simulink model "sim_tvt_2025_pos_ctrl"  (R2020a)
settings: Solver=ode4  StartTime=0.0  StopTime=30.0  FixedStep=0.01  RelTol=1e-3
values from neighbouring files (symbols this model uses):
  alfa = 0.02    [init_tvt_2025_pos_ctrl.m]
  alfa_theta = 20    [init_tvt_2025_pos_ctrl.m]
  alfa_theta_obs = 100    [init_tvt_2025_pos_ctrl.m]
  c0 = 0.1    [init_tvt_2025_pos_ctrl.m]
  c1_diff_sigma_bar_v = diag([25; 30; 20])    [init_tvt_2025_pos_ctrl.m]
  c1v = diag([5.8; 6.5; 6.5])    [init_tvt_2025_pos_ctrl.m]
  c2_diff_sigma_bar_v = diag([50; 50; 10])    [init_tvt_2025_pos_ctrl.m]
  c2v = diag([5.8; 6.5; 6.5])    [init_tvt_2025_pos_ctrl.m]
  c3_diff_sigma_bar_v = diag([15; 15; 10])    [init_tvt_2025_pos_ctrl.m]
  c3v = diag([4.8; 6.4; 6.0])    [init_tvt_2025_pos_ctrl.m]
  delta_p_i_0 = zeros(3, NF)    [init_tvt_2025_pos_ctrl.m]
  delta_v_i_0 = zeros(3, NF)    [init_tvt_2025_pos_ctrl.m]
  dp_aa_t = 0.2 * ones(3, 5) + ( 1.0 - 0.2 ) * rand(3, 5)    [init_tvt_2025_pos_ctrl.m]
  dp_ff_t = [ 0.4 * ones(1, 5) + ( 1.0 - 0.4 ) * rand(1, 5);                      0.4 * ones(1, 5) + ( 1.0 - 0.4 ) * rand(1, 5);                      0.2 * ones(1, 5) + ( 0.6 - 0.2 ) * rand(1, 5) ]    [init_tvt_2025_pos_ctrl.m]
  dp_phi_t = ( - pi / 2 ) * ones(3, 5) + ( pi / 2 - ( - pi / 2 ) ) * rand(3, 5)    [init_tvt_2025_pos_ctrl.m]
  eps0 = [0.05; 0.01; 0.01]    [init_tvt_2025_pos_ctrl.m]
  eta_ld_hat_init = zeros(3,NF)    [init_tvt_2025_pos_ctrl.m]
  etai_0 = zeros(3,5)    [init_tvt_2025_pos_ctrl.m]
  gamma0 = diag([1, 1, 1])    [init_tvt_2025_pos_ctrl.m]
  k_phi = diag([10, 10, 10])    [init_tvt_2025_pos_ctrl.m]
  k_theta = diag([5, 5, 5])    [init_tvt_2025_pos_ctrl.m]
  kai0 = [15; 10; 10]    [init_tvt_2025_pos_ctrl.m]
  kai_1_t = 0.02    [init_tvt_2025_pos_ctrl.m]
  kai_3_t = 0.1    [init_tvt_2025_pos_ctrl.m]
  ksi_ld_hat_init = zeros(3,NF)    [init_tvt_2025_pos_ctrl.m]
  ksii_0 = zeros(3,5)    [init_tvt_2025_pos_ctrl.m]
  l1v = diag([20; 20; 20])    [init_tvt_2025_pos_ctrl.m]
  l2v = diag([30; 30; 30])    [init_tvt_2025_pos_ctrl.m]
  lam0 = [15; 10; 10]    [init_tvt_2025_pos_ctrl.m]
  lam1 = diag([5,5,5])    [init_tvt_2025_pos_ctrl.m]
  lam2 = diag([5,5,5])    [init_tvt_2025_pos_ctrl.m]
  lam3 = diag([5,5,5])    [init_tvt_2025_pos_ctrl.m]
  lam4 = diag([5,5,5])    [init_tvt_2025_pos_ctrl.m]
  Lamd_diff_sigma_bar_v = 0.5    [init_tvt_2025_pos_ctrl.m]
  mass_i = zeros(1,NF)    [init_tvt_2025_pos_ctrl.m]
  Mii = diag([1;0;0;0;1])    [init_tvt_2025_pos_ctrl.m]
  pos0 = zeros(3, 1)    [init_tvt_2025_pos_ctrl.m]
  pos_bar_init = zeros(3,NF)    [init_tvt_2025_pos_ctrl.m]
  PZ0 = P0(3)    [init_tvt_2025_pos_ctrl.m]
  PZ1 = 10    [init_tvt_2025_pos_ctrl.m]
  Qci_init = repmat([1;0;0;0],1,NF)    [init_tvt_2025_pos_ctrl.m]
  R0 = 4    [init_tvt_2025_pos_ctrl.m]
  R1 = 8    [init_tvt_2025_pos_ctrl.m]
  Rx2 = 10    [init_tvt_2025_pos_ctrl.m]
  Ry2 = 6    [init_tvt_2025_pos_ctrl.m]
  Rz2 = 4    [init_tvt_2025_pos_ctrl.m]
  T0 = 0    [init_tvt_2025_pos_ctrl.m]
  T1 = tseq1    (= 10)    [init_tvt_2025_pos_ctrl.m]
  T12 = tseq1 + tseq12    (= 20)    [init_tvt_2025_pos_ctrl.m]
  T2 = tseq1 + tseq12 + tseq2    (= 30)    [init_tvt_2025_pos_ctrl.m]
  theta0 = ( 2 / 5 ) * pi    (= 1.25663706144)    [init_tvt_2025_pos_ctrl.m]
  vel0 = zeros(3, 1)    [init_tvt_2025_pos_ctrl.m]
  vel_bar_init = zeros(3,NF)    [init_tvt_2025_pos_ctrl.m]
  Wij = [0,0,1,0,0;              0,0,1,1,0;              1,0,0,0,1;              0,1,1,0,0;              0,0,1,0,0]    [init_tvt_2025_pos_ctrl.m]
  X1 = 8    [init_tvt_2025_pos_ctrl.m]
  X2 = 2    [init_tvt_2025_pos_ctrl.m]
  X3 = 3    [init_tvt_2025_pos_ctrl.m]
  Y1 = 10    [init_tvt_2025_pos_ctrl.m]
  Y2 = 2    [init_tvt_2025_pos_ctrl.m]
  Y3 = 4    [init_tvt_2025_pos_ctrl.m]
  Z1 = 4    [init_tvt_2025_pos_ctrl.m]
  Z2 = -6    [init_tvt_2025_pos_ctrl.m]
  Z3 = 2    [init_tvt_2025_pos_ctrl.m]
  zeta_diff_sigma_bar_v = 0.08    [init_tvt_2025_pos_ctrl.m]
undefined symbols (not defined in the file or in its folder): cal_frac_squ, p_alfav1, p_alfav2, p_gamma1_pos, p_gamma1_vel, p_gamma2_pos, p_gamma2_vel, q_alfav1, q_alfav2, q_gamma1_pos, q_gamma1_vel, q_gamma2_pos, q_gamma2_vel
(part 5 of 5)

== matlab function sim_tvt_2025_pos_ctrl/combine lumped follower position observation error ==
  data: theta_ksi_est_err_tilt_1_1 input; theta_ksi_est_err_tilt_1_2 input; theta_ksi_est_err_tilt_1_3 input; theta_ksi_est_err_tilt_1_4 input; theta_ksi_est_err_tilt_1_5 input; theta_ksi_est_err_tilt_1_vec output; theta_ksi_est_err_tilt_2_1 input; theta_ksi_est_err_tilt_2_vec output; theta_ksi_est_err_tilt_2_2 input; theta_ksi_est_err_tilt_2_3 input; theta_ksi_est_err_tilt_2_4 input; theta_ksi_est_err_tilt_2_5 input
function [theta_ksi_est_err_tilt_1_vec, theta_ksi_est_err_tilt_2_vec]  = fcn(theta_ksi_est_err_tilt_1_1, theta_ksi_est_err_tilt_1_2, theta_ksi_est_err_tilt_1_3, theta_ksi_est_err_tilt_1_4, theta_ksi_est_err_tilt_1_5, ...
                                                                                                                                    theta_ksi_est_err_tilt_2_1, theta_ksi_est_err_tilt_2_2, theta_ksi_est_err_tilt_2_3, theta_ksi_est_err_tilt_2_4, theta_ksi_est_err_tilt_2_5)
%%%% 合并领导者位置观测器输出结果
theta_ksi_est_err_tilt_1_vec = [theta_ksi_est_err_tilt_1_1(:), theta_ksi_est_err_tilt_1_2(:), theta_ksi_est_err_tilt_1_3(:), theta_ksi_est_err_tilt_1_4(:), theta_ksi_est_err_tilt_1_5(:)];
theta_ksi_est_err_tilt_2_vec = [theta_ksi_est_err_tilt_2_1(:), theta_ksi_est_err_tilt_2_2(:), theta_ksi_est_err_tilt_2_3(:), theta_ksi_est_err_tilt_2_4(:), theta_ksi_est_err_tilt_2_5(:)];

== matlab function sim_tvt_2025_pos_ctrl/cal rho_err_vec ==
  data: u0 input; rho_err_vec output; rho_hat_vec input
function rho_err_vec  = fcn(u0, rho_hat_vec)
%%%% 计算分布式观测误差
rho_err_vec = zeros(3,5);
for iiuav = 1:5
    rho_err_vec(:,iiuav) = u0(:) - rho_hat_vec(:,iiuav);
end

== matlab function sim_tvt_2025_pos_ctrl/combine lumped follower velocity observation error ==
  data: theta_eta_est_err_tilt_1_1 input; theta_eta_est_err_tilt_1_2 input; theta_eta_est_err_tilt_1_3 input; theta_eta_est_err_tilt_1_4 input; theta_eta_est_err_tilt_1_5 input; theta_eta_est_err_tilt_1_vec output; theta_eta_est_err_tilt_2_1 input; theta_eta_est_err_tilt_2_vec output; theta_eta_est_err_tilt_2_2 input; theta_eta_est_err_tilt_2_3 input; theta_eta_est_err_tilt_2_4 input; theta_eta_est_err_tilt_2_5 input
function [theta_eta_est_err_tilt_1_vec, theta_eta_est_err_tilt_2_vec]  = fcn(theta_eta_est_err_tilt_1_1, theta_eta_est_err_tilt_1_2, theta_eta_est_err_tilt_1_3, theta_eta_est_err_tilt_1_4, theta_eta_est_err_tilt_1_5, ...
                                                                                                                                    theta_eta_est_err_tilt_2_1, theta_eta_est_err_tilt_2_2, theta_eta_est_err_tilt_2_3, theta_eta_est_err_tilt_2_4, theta_eta_est_err_tilt_2_5)
%%%% 合并领导者位置观测器输出结果
theta_eta_est_err_tilt_1_vec = [theta_eta_est_err_tilt_1_1(:), theta_eta_est_err_tilt_1_2(:), theta_eta_est_err_tilt_1_3(:), theta_eta_est_err_tilt_1_4(:), theta_eta_est_err_tilt_1_5(:)];
theta_eta_est_err_tilt_2_vec = [theta_eta_est_err_tilt_2_1(:), theta_eta_est_err_tilt_2_2(:), theta_eta_est_err_tilt_2_3(:), theta_eta_est_err_tilt_2_4(:), theta_eta_est_err_tilt_2_5(:)];

== matlab function sim_tvt_2025_pos_ctrl/fixed-time distributed follower desire position observer agent 1 ==
  data: l1p input; d_ksi_d_est_1 output; l2p input; eta_d_est_vec input; theta_ksi_est_err_tilt_1_vec input; theta_ksi_est_err_tilt_2_vec input
function d_ksi_d_est_1 = fcn(l1p, l2p, eta_d_est_vec, theta_ksi_est_err_tilt_1_vec, theta_ksi_est_err_tilt_2_vec)
%%%% 固定时间跟随者期望位置分布式观测器
iiuav = 1;
d_ksi_d_est_1 = eta_d_est_vec(:,iiuav) - l1p * theta_ksi_est_err_tilt_1_vec(:,iiuav) - l2p * theta_ksi_est_err_tilt_2_vec(:,iiuav);

== matlab function sim_tvt_2025_pos_ctrl/fixed-time distributed follower desire position observer agent 2 ==
  data: l1p input; d_ksi_d_est_2 output; l2p input; eta_d_est_vec input; theta_ksi_est_err_tilt_1_vec input; theta_ksi_est_err_tilt_2_vec input
function d_ksi_d_est_2 = fcn(l1p, l2p, eta_d_est_vec, theta_ksi_est_err_tilt_1_vec, theta_ksi_est_err_tilt_2_vec)
%%%% 固定时间跟随者期望位置分布式观测器
iiuav = 2;
d_ksi_d_est_2 = eta_d_est_vec(:,iiuav) - l1p * theta_ksi_est_err_tilt_1_vec(:,iiuav) - l2p * theta_ksi_est_err_tilt_2_vec(:,iiuav);

== matlab function sim_tvt_2025_pos_ctrl/fixed-time distributed follower desire position observer agent 3 ==
  data: l1p input; d_ksi_d_est_3 output; l2p input; eta_d_est_vec input; theta_ksi_est_err_tilt_1_vec input; theta_ksi_est_err_tilt_2_vec input
function d_ksi_d_est_3 = fcn(l1p, l2p, eta_d_est_vec, theta_ksi_est_err_tilt_1_vec, theta_ksi_est_err_tilt_2_vec)
%%%% 固定时间跟随者期望位置分布式观测器
iiuav = 3;
d_ksi_d_est_3 = eta_d_est_vec(:,iiuav) - l1p * theta_ksi_est_err_tilt_1_vec(:,iiuav) - l2p * theta_ksi_est_err_tilt_2_vec(:,iiuav);

== matlab function sim_tvt_2025_pos_ctrl/fixed-time distributed follower desire position observer agent 4 ==
  data: l1p input; d_ksi_d_est_4 output; l2p input; eta_d_est_vec input; theta_ksi_est_err_tilt_1_vec input; theta_ksi_est_err_tilt_2_vec input
function d_ksi_d_est_4 = fcn(l1p, l2p, eta_d_est_vec, theta_ksi_est_err_tilt_1_vec, theta_ksi_est_err_tilt_2_vec)
%%%% 固定时间跟随者期望位置分布式观测器
iiuav = 4;
d_ksi_d_est_4 = eta_d_est_vec(:,iiuav) - l1p * theta_ksi_est_err_tilt_1_vec(:,iiuav) - l2p * theta_ksi_est_err_tilt_2_vec(:,iiuav);

== matlab function sim_tvt_2025_pos_ctrl/fixed-time distributed follower desire position observer agent 5 ==
  data: l1p input; d_ksi_d_est_5 output; l2p input; eta_d_est_vec input; theta_ksi_est_err_tilt_1_vec input; theta_ksi_est_err_tilt_2_vec input
function d_ksi_d_est_5 = fcn(l1p, l2p, eta_d_est_vec, theta_ksi_est_err_tilt_1_vec, theta_ksi_est_err_tilt_2_vec)
%%%% 固定时间跟随者期望位置分布式观测器
iiuav = 5;
d_ksi_d_est_5 = eta_d_est_vec(:,iiuav) - l1p * theta_ksi_est_err_tilt_1_vec(:,iiuav) - l2p * theta_ksi_est_err_tilt_2_vec(:,iiuav);

== matlab function sim_tvt_2025_pos_ctrl/fixed-time distributed follower desire velocity observer agent 1 ==
  data: l1v input; d_eta_d_est_1 output; l2v input; theta_eta_est_err_tilt_1_vec input; theta_eta_est_err_tilt_2_vec input
function d_eta_d_est_1 = fcn(l1v, l2v, theta_eta_est_err_tilt_1_vec, theta_eta_est_err_tilt_2_vec)
%%%% 固定时间跟随者期望速度分布式观测器
iiuav = 1;
d_eta_d_est_1 = -l1v * theta_eta_est_err_tilt_1_vec(:,iiuav) - l2v * theta_eta_est_err_tilt_2_vec(:,iiuav);

== matlab function sim_tvt_2025_pos_ctrl/cal abs 41 ==
  data: x input; y output
function y = fcn(x)
y = abs(x(:));

== matlab function sim_tvt_2025_pos_ctrl/fixed-time distributed follower desire velocity observer agent 2 ==
  data: l1v input; d_eta_d_est_2 output; l2v input; theta_eta_est_err_tilt_1_vec input; theta_eta_est_err_tilt_2_vec input
function d_eta_d_est_2 = fcn(l1v, l2v, theta_eta_est_err_tilt_1_vec, theta_eta_est_err_tilt_2_vec)
%%%% 固定时间跟随者期望速度分布式观测器
iiuav = 2;
d_eta_d_est_2 = -l1v * theta_eta_est_err_tilt_1_vec(:,iiuav) - l2v * theta_eta_est_err_tilt_2_vec(:,iiuav);

== matlab function sim_tvt_2025_pos_ctrl/fixed-time distributed follower desire velocity observer agent 3 ==
  data: l1v input; d_eta_d_est_3 output; l2v input; theta_eta_est_err_tilt_1_vec input; theta_eta_est_err_tilt_2_vec input
function d_eta_d_est_3 = fcn(l1v, l2v, theta_eta_est_err_tilt_1_vec, theta_eta_est_err_tilt_2_vec)
%%%% 固定时间跟随者期望速度分布式观测器
iiuav = 3;
d_eta_d_est_3 = -l1v * theta_eta_est_err_tilt_1_vec(:,iiuav) - l2v * theta_eta_est_err_tilt_2_vec(:,iiuav);

== matlab function sim_tvt_2025_pos_ctrl/fixed-time distributed follower desire velocity observer agent 4 ==
  data: l1v input; d_eta_d_est_4 output; l2v input; theta_eta_est_err_tilt_1_vec input; theta_eta_est_err_tilt_2_vec input
function d_eta_d_est_4 = fcn(l1v, l2v, theta_eta_est_err_tilt_1_vec, theta_eta_est_err_tilt_2_vec)
%%%% 固定时间跟随者期望速度分布式观测器
iiuav = 4;
d_eta_d_est_4 = -l1v * theta_eta_est_err_tilt_1_vec(:,iiuav) - l2v * theta_eta_est_err_tilt_2_vec(:,iiuav);

== matlab function sim_tvt_2025_pos_ctrl/fixed-time distributed follower desire velocity observer agent 5 ==
  data: l1v input; d_eta_d_est_5 output; l2v input; theta_eta_est_err_tilt_1_vec input; theta_eta_est_err_tilt_2_vec input
function d_eta_d_est_5 = fcn(l1v, l2v, theta_eta_est_err_tilt_1_vec, theta_eta_est_err_tilt_2_vec)
%%%% 固定时间跟随者期望速度分布式观测器
iiuav = 5;
d_eta_d_est_5 = -l1v * theta_eta_est_err_tilt_1_vec(:,iiuav) - l2v * theta_eta_est_err_tilt_2_vec(:,iiuav);

== matlab function sim_tvt_2025_pos_ctrl/trans to column41 ==
  data: x input; y output
function y = fcn(x)
y = x(:);

== matlab function sim_tvt_2025_pos_ctrl/trans to column42 ==
  data: x input; y output
function y = fcn(x)
y = x(:);

== matlab function sim_tvt_2025_pos_ctrl/trans to column43 ==
  data: x input; y output
function y = fcn(x)
y = x(:);

== matlab function sim_tvt_2025_pos_ctrl/trans to column44 ==
  data: x input; y output
function y = fcn(x)
y = x(:);

== matlab function sim_tvt_2025_pos_ctrl/cal abs 42 ==
  data: x input; y output
function y = fcn(x)
y = abs(x(:));

== matlab function sim_tvt_2025_pos_ctrl/trans to column45 ==
  data: x input; y output
function y = fcn(x)
y = x(:);

== matlab function sim_tvt_2025_pos_ctrl/trans to column46 ==
  data: x input; y output
function y = fcn(x)
y = x(:);

== matlab function sim_tvt_2025_pos_ctrl/trans to column47 ==
  data: x input; y output
function y = fcn(x)
y = x(:);

== matlab function sim_tvt_2025_pos_ctrl/trans to column48 ==
  data: x input; y output
function y = fcn(x)
y = x(:);

== matlab function sim_tvt_2025_pos_ctrl/trans to column49 ==
  data: x input; y output
function y = fcn(x)
y = x(:);

== matlab function sim_tvt_2025_pos_ctrl/trans to column50 ==
  data: x input; y output
function y = fcn(x)
y = x(:);

== matlab function sim_tvt_2025_pos_ctrl/trans to column51 ==
  data: x input; y output
function y = fcn(x)
y = x(:);

== matlab function sim_tvt_2025_pos_ctrl/trans to column52 ==
  data: x input; y output
function y = fcn(x)
y = x(:);

== matlab function sim_tvt_2025_pos_ctrl/trans to column53 ==
  data: x input; y output
function y = fcn(x)
y = x(:);

== matlab function sim_tvt_2025_pos_ctrl/trans to column54 ==
  data: x input; y output
function y = fcn(x)
y = x(:);

== matlab function sim_tvt_2025_pos_ctrl/cal abs 43 ==
  data: x input; y output
function y = fcn(x)
y = abs(x(:));

== matlab function sim_tvt_2025_pos_ctrl/trans to column55 ==
  data: x input; y output
function y = fcn(x)
y = x(:);

== matlab function sim_tvt_2025_pos_ctrl/trans to column56 ==
  data: x input; y output
function y = fcn(x)
y = x(:);

== matlab function sim_tvt_2025_pos_ctrl/trans to column57 ==
  data: x input; y output
function y = fcn(x)
y = x(:);

== matlab function sim_tvt_2025_pos_ctrl/trans to column58 ==
  data: x input; y output
function y = fcn(x)
y = x(:);

== matlab function sim_tvt_2025_pos_ctrl/trans to column59 ==
  data: x input; y output
function y = fcn(x)
y = x(:);

== matlab function sim_tvt_2025_pos_ctrl/trans to column60 ==
  data: x input; y output
function y = fcn(x)
y = x(:);

== matlab function sim_tvt_2025_pos_ctrl/cal abs 44 ==
  data: x input; y output
function y = fcn(x)
y = abs(x(:));

== matlab function sim_tvt_2025_pos_ctrl/cal abs 45 ==
  data: x input; y output
function y = fcn(x)
y = abs(x(:));

== matlab function sim_tvt_2025_pos_ctrl/cal ui agent 2 ==
  data: k_phi input; rho_hat_vec input; phi_vec input; d_phi_vec input; ui_2 output; dp_hat_vec input
function ui_2 = fcn(k_phi, rho_hat_vec, phi_vec, d_phi_vec, dp_hat_vec)
%%%% 计算控制输入ui
iiuav = 2;
g0 = 9.80663;
e3 = [0;0;1];
ui_2 = g0 * e3 + rho_hat_vec(:,iiuav) - dp_hat_vec(:,iiuav) ...
            - k_phi * ( tanh( phi_vec(:,iiuav) ) + tanh( d_phi_vec(:,iiuav) ) );

== matlab function sim_tvt_2025_pos_ctrl/cal ui agent 3 ==
  data: k_phi input; rho_hat_vec input; phi_vec input; d_phi_vec input; ui_3 output; dp_hat_vec input
function ui_3 = fcn(k_phi, rho_hat_vec, phi_vec, d_phi_vec, dp_hat_vec)
%%%% 计算控制输入ui
iiuav = 3;
g0 = 9.80663;
e3 = [0;0;1];
ui_3 = g0 * e3 + rho_hat_vec(:,iiuav) - dp_hat_vec(:,iiuav) ...
            - k_phi * ( tanh( phi_vec(:,iiuav) ) + tanh( d_phi_vec(:,iiuav) ) );

== matlab function sim_tvt_2025_pos_ctrl/cal ui agent 4 ==
  data: k_phi input; rho_hat_vec input; phi_vec input; d_phi_vec input; ui_4 output; dp_hat_vec input
function ui_4 = fcn(k_phi, rho_hat_vec, phi_vec, d_phi_vec, dp_hat_vec)
%%%% 计算控制输入ui
iiuav = 4;
g0 = 9.80663;
e3 = [0;0;1];
ui_4 = g0 * e3 + rho_hat_vec(:,iiuav) - dp_hat_vec(:,iiuav) ...
            - k_phi * ( tanh( phi_vec(:,iiuav) ) + tanh( d_phi_vec(:,iiuav) ) );

== matlab function sim_tvt_2025_pos_ctrl/cal ui agent 5 ==
  data: k_phi input; rho_hat_vec input; phi_vec input; d_phi_vec input; ui_5 output; dp_hat_vec input
function ui_5 = fcn(k_phi, rho_hat_vec, phi_vec, d_phi_vec, dp_hat_vec)
%%%% 计算控制输入ui
iiuav = 5;
g0 = 9.80663;
e3 = [0;0;1];
ui_5 = g0 * e3 + rho_hat_vec(:,iiuav) - dp_hat_vec(:,iiuav) ...
            - k_phi * ( tanh( phi_vec(:,iiuav) ) + tanh( d_phi_vec(:,iiuav) ) );

== matlab function sim_tvt_2025_pos_ctrl/cal abs 46 ==
  data: x input; y output
function y = fcn(x)
y = abs(x(:));

== matlab function sim_tvt_2025_pos_ctrl/combine formation control input ==
  data: eta_i_vec output; ksi_i_vec output; eta_1 input; eta_2 input; eta_3 input; eta_4 input; eta_5 input; ksi_1 input; ksi_2 input; ksi_3 input; ksi_4 input; ksi_5 input
function [eta_i_vec, ksi_i_vec] = fcn(eta_1, eta_2, eta_3, eta_4, eta_5, ...
                                                                ksi_1, ksi_2, ksi_3, ksi_4, ksi_5)
%%%% 合并领导者编队跟踪误差结果
eta_i_vec = [eta_1(:), eta_2(:), eta_3(:), eta_4(:), eta_5(:)];
ksi_i_vec = [ksi_1(:), ksi_2(:), ksi_3(:), ksi_4(:), ksi_5(:)];

== matlab function sim_tvt_2025_pos_ctrl/cal abs 47 ==
  data: x input; y output
function y = fcn(x)
y = abs(x(:));

== matlab function sim_tvt_2025_pos_ctrl/cal abs 48 ==
  data: x input; y output
function y = fcn(x)
y = abs(x(:));

== matlab function sim_tvt_2025_pos_ctrl/cal abs 49 ==
  data: x input; y output
function y = fcn(x)
y = abs(x(:));

== matlab function sim_tvt_2025_pos_ctrl/cal abs 50 ==
  data: x input; y output
function y = fcn(x)
y = abs(x(:));

== matlab function sim_tvt_2025_pos_ctrl/uav translational dynamics agent 1 ==
  data: dvi output; Ri input; ui input; dpi_vec input
function dvi = fcn(Ri, ui, dpi_vec)
%%%% 根据有限时间控制输入计算无人机平移动力学微分方程
iiuav = 1;
g0 = 9.80663;
e3 = [0;0;1];
dvi = -g0 * e3 + norm(ui(:,iiuav),2) * Ri(:,:,iiuav) * e3 + dpi_vec(:,iiuav);

== matlab function sim_tvt_2025_pos_ctrl/uav translational dynamics agent 2 ==
  data: dvi output; Ri input; ui input; dpi_vec input
function dvi = fcn(Ri, ui, dpi_vec)
%%%% 根据有限时间控制输入计算无人机平移动力学微分方程
iiuav = 2;
g0 = 9.80663;
e3 = [0;0;1];
dvi = -g0 * e3 + norm(ui(:,iiuav),2) * Ri(:,:,iiuav) * e3 + dpi_vec(:,iiuav);

== matlab function sim_tvt_2025_pos_ctrl/uav translational dynamics agent 3 ==
  data: dvi output; Ri input; ui input; dpi_vec input
function dvi = fcn(Ri, ui, dpi_vec)
%%%% 根据有限时间控制输入计算无人机平移动力学微分方程
iiuav = 3;
g0 = 9.80663;
e3 = [0;0;1];
dvi = -g0 * e3 + norm(ui(:,iiuav),2) * Ri(:,:,iiuav) * e3 + dpi_vec(:,iiuav);

== matlab function sim_tvt_2025_pos_ctrl/uav translational dynamics agent 4 ==
  data: dvi output; Ri input; ui input; dpi_vec input
function dvi = fcn(Ri, ui, dpi_vec)
%%%% 根据有限时间控制输入计算无人机平移动力学微分方程
iiuav = 4;
g0 = 9.80663;
e3 = [0;0;1];
dvi = -g0 * e3 + norm(ui(:,iiuav),2) * Ri(:,:,iiuav) * e3 + dpi_vec(:,iiuav);

== matlab function sim_tvt_2025_pos_ctrl/uav translational dynamics agent 5 ==
  data: dvi output; Ri input; ui input; dpi_vec input
function dvi = fcn(Ri, ui, dpi_vec)
%%%% 根据有限时间控制输入计算无人机平移动力学微分方程
iiuav = 5;
g0 = 9.80663;
e3 = [0;0;1];
dvi = -g0 * e3 + norm(ui(:,iiuav),2) * Ri(:,:,iiuav) * e3 + dpi_vec(:,iiuav);

== matlab function sim_tvt_2025_pos_ctrl/cal Ri ==
  data: Ri output; Rei input; Rci input
function Ri = fcn(Rei, Rci)
%%%% 使用罗德里格公式由四元数Qci求解Rci
Ri = zeros(3,3,5);
for iiuav = 1:5
    Ri(:,:,iiuav) = Rci(:,:,iiuav) * Rei(:,:,iiuav);
end

end

== matlab function sim_tvt_2025_pos_ctrl/follower tracking error agent 1 ==
  data: ksi_track_err_1 output; delta_ksi_vec input; delta_eta_vec input; ksi_i_vec input; eta_i_vec input; ksi0 input; eta_track_err_1 output; eta0 input
function [ksi_track_err_1, eta_track_err_1]  = fcn(delta_ksi_vec, delta_eta_vec, ksi_i_vec, eta_i_vec, ksi0, eta0)
%%%% 计算跟随者节点1号位置/速度跟踪误差
eta_track_err_1 = eta_i_vec(:,1) - delta_eta_vec(:,1) - eta0;
ksi_track_err_1 = ksi_i_vec(:,1) - delta_ksi_vec(:,1) - ksi0;

== matlab function sim_tvt_2025_pos_ctrl/follower tracking error agent 2 ==
  data: ksi_track_err_2 output; delta_ksi_vec input; delta_eta_vec input; ksi_i_vec input; eta_i_vec input; ksi0 input; eta_track_err_2 output; eta0 input
function [ksi_track_err_2, eta_track_err_2]  = fcn(delta_ksi_vec, delta_eta_vec, ksi_i_vec, eta_i_vec, ksi0, eta0)
%%%% 计算跟随者节点2号位置/速度跟踪误差
eta_track_err_2 = eta_i_vec(:,2) - delta_eta_vec(:,2) - eta0;
ksi_track_err_2 = ksi_i_vec(:,2) - delta_ksi_vec(:,2) - ksi0;

== matlab function sim_tvt_2025_pos_ctrl/follower tracking error agent 3 ==
  data: ksi_track_err_3 output; delta_ksi_vec input; delta_eta_vec input; ksi_i_vec input; eta_i_vec input; ksi0 input; eta_track_err_3 output; eta0 input
function [ksi_track_err_3, eta_track_err_3]  = fcn(delta_ksi_vec, delta_eta_vec, ksi_i_vec, eta_i_vec, ksi0, eta0)
%%%% 计算跟随者节点3号位置/速度跟踪误差
eta_track_err_3 = eta_i_vec(:,3) - delta_eta_vec(:,3) - eta0;
ksi_track_err_3 = ksi_i_vec(:,3) - delta_ksi_vec(:,3) - ksi0;

== matlab function sim_tvt_2025_pos_ctrl/follower tracking error agent 4 ==
  data: ksi_track_err_4 output; delta_ksi_vec input; delta_eta_vec input; ksi_i_vec input; eta_i_vec input; ksi0 input; eta_track_err_4 output; eta0 input
function [ksi_track_err_4, eta_track_err_4]  = fcn(delta_ksi_vec, delta_eta_vec, ksi_i_vec, eta_i_vec, ksi0, eta0)
%%%% 计算跟随者节点4号位置/速度跟踪误差
eta_track_err_4 = eta_i_vec(:,4) - delta_eta_vec(:,4) - eta0;
ksi_track_err_4 = ksi_i_vec(:,4) - delta_ksi_vec(:,4) - ksi0;

== matlab function sim_tvt_2025_pos_ctrl/follower tracking error agent 5 ==
  data: ksi_track_err_5 output; delta_ksi_vec input; delta_eta_vec input; ksi_i_vec input; eta_i_vec input; ksi0 input; eta_track_err_5 output; eta0 input
function [ksi_track_err_5, eta_track_err_5]  = fcn(delta_ksi_vec, delta_eta_vec, ksi_i_vec, eta_i_vec, ksi0, eta0)
%%%% 计算跟随者节点5号位置/速度跟踪误差
eta_track_err_5 = eta_i_vec(:,5) - delta_eta_vec(:,5) - eta0;
ksi_track_err_5 = ksi_i_vec(:,5) - delta_ksi_vec(:,5) - ksi0;

== matlab function sim_tvt_2025_pos_ctrl/combine follower eta ksi ==
  data: ksi_track_err_vec output; ksi_track_err_1 input; ksi_track_err_2 input; ksi_track_err_3 input; ksi_track_err_4 input; ksi_track_err_5 input; eta_track_err_vec output; eta_track_err_1 input; eta_track_err_2 input; eta_track_err_3 input; eta_track_err_4 input; eta_track_err_5 input
function [ksi_track_err_vec, eta_track_err_vec]  = fcn(ksi_track_err_1, ksi_track_err_2, ksi_track_err_3, ksi_track_err_4, ksi_track_err_5, ...
                                                                                    eta_track_err_1, eta_track_err_2, eta_track_err_3, eta_track_err_4, eta_track_err_5)
%%%% 合并所有跟随者的速度/位置向量
ksi_track_err_vec = [ksi_track_err_1(:), ksi_track_err_2(:), ksi_track_err_3(:), ksi_track_err_4(:), ksi_track_err_5(:)];
eta_track_err_vec = [eta_track_err_1(:), eta_track_err_2(:), eta_track_err_3(:), eta_track_err_4(:), eta_track_err_5(:)];

== matlab function sim_tvt_2025_pos_ctrl/depart Rc5 ==
  data: y output; x input
function y = fcn(x)
y = x(:,:,5);

end

== matlab function sim_tvt_2025_pos_ctrl/depart Rc1 ==
  data: y output; x input
function y = fcn(x)
y = x(:,:,1);

end

== matlab function sim_tvt_2025_pos_ctrl/depart Rc2 ==
  data: y output; x input
function y = fcn(x)
y = x(:,:,2);

end

== matlab function sim_tvt_2025_pos_ctrl/depart Rc3 ==
  data: y output; x input
function y = fcn(x)
y = x(:,:,3);

end

== matlab function sim_tvt_2025_pos_ctrl/depart Rc4 ==
  data: y output; x input
function y = fcn(x)
y = x(:,:,4);

end

== matlab function sim_tvt_2025_pos_ctrl/combine rho_hat ==
  data: rho_hat_1 input; rho_hat_vec output; rho_hat_2 input; rho_hat_3 input; rho_hat_4 input; rho_hat_5 input
function rho_hat_vec  = fcn(rho_hat_1, rho_hat_2, rho_hat_3, rho_hat_4, rho_hat_5)
%%%% 合并领导者加速度分布式观测器
rho_hat_vec = zeros(3,5);
rho_hat_vec(:,1) = rho_hat_1(:);
rho_hat_vec(:,2) = rho_hat_2(:);
rho_hat_vec(:,3) = rho_hat_3(:);
rho_hat_vec(:,4) = rho_hat_4(:);
rho_hat_vec(:,5) = rho_hat_5(:);

== matlab function sim_tvt_2025_pos_ctrl/rho_hat agent 1 ==
  data: lam0 input; rho_hat_1 output; sigmai_vec input
function rho_hat_1 = fcn(lam0, sigmai_vec)
%%%% 领导者加速度分布式观测器
iiuav = 1;
rho_hat_1 = lam0(:) .* tanh( sigmai_vec(:,iiuav) );

== matlab function sim_tvt_2025_pos_ctrl/rho_hat agent 2 ==
  data: lam0 input; rho_hat_2 output; sigmai_vec input
function rho_hat_2 = fcn(lam0, sigmai_vec)
%%%% 领导者加速度分布式观测器
iiuav = 2;
rho_hat_2 = lam0(:) .* tanh( sigmai_vec(:,iiuav) );

== matlab function sim_tvt_2025_pos_ctrl/rho_hat agent 3 ==
  data: lam0 input; rho_hat_3 output; sigmai_vec input
function rho_hat_3 = fcn(lam0, sigmai_vec)
%%%% 领导者加速度分布式观测器
iiuav = 3;
rho_hat_3 = lam0(:) .* tanh( sigmai_vec(:,iiuav) );

== matlab function sim_tvt_2025_pos_ctrl/rho_hat agent 4 ==
  data: lam0 input; rho_hat_4 output; sigmai_vec input
function rho_hat_4 = fcn(lam0, sigmai_vec)
%%%% 领导者加速度分布式观测器
iiuav = 4;
rho_hat_4 = lam0(:) .* tanh( sigmai_vec(:,iiuav) );

== matlab function sim_tvt_2025_pos_ctrl/rho_hat agent 5 ==
  data: lam0 input; rho_hat_5 output; sigmai_vec input
function rho_hat_5 = fcn(lam0, sigmai_vec)
%%%% 领导者加速度分布式观测器
iiuav = 5;
rho_hat_5 = lam0(:) .* tanh( sigmai_vec(:,iiuav) );

== matlab function sim_tvt_2025_pos_ctrl/cal abs 51 ==
  data: x input; y output
function y = fcn(x)
y = abs(x(:));

== matlab function sim_tvt_2025_pos_ctrl/cal abs 52 ==
  data: x input; y output
function y = fcn(x)
y = abs(x(:));

== matlab function sim_tvt_2025_pos_ctrl/cal abs 53 ==
  data: x input; y output
function y = fcn(x)
y = abs(x(:));

== matlab function sim_tvt_2025_pos_ctrl/cal abs 54 ==
  data: x input; y output
function y = fcn(x)
y = abs(x(:));

== matlab function sim_tvt_2025_pos_ctrl/cal abs 55 ==
  data: x input; y output
function y = fcn(x)
y = abs(x(:));

== matlab function sim_tvt_2025_pos_ctrl/cal leader velocity estimate error ==
  data: eta_ld_hat_vec input; eta_ld_est_err output; eta0 input
function eta_ld_est_err  = fcn(eta_ld_hat_vec, eta0)
%%%% 计算领导者速度分布式观测误差
eta_ld_est_err = zeros(3,5);
for iiuav = 1:5
    eta_ld_est_err(:,iiuav) = eta_ld_hat_vec(:,iiuav) - eta0(:);
end

== matlab function sim_tvt_2025_pos_ctrl/cal leader position estimate error ==
  data: ksi_ld_hat_vec input; ksi_ld_est_err output; ksi0 input
function ksi_ld_est_err  = fcn(ksi_ld_hat_vec, ksi0)
%%%% 计算领导者位置分布式观测误差
ksi_ld_est_err = zeros(3,5);
for iiuav = 1:5
    ksi_ld_est_err(:,iiuav) = ksi_ld_hat_vec(:,iiuav) - ksi0(:);
end

== matlab function sim_tvt_2025_pos_ctrl/generate translational disturbance agent 1 ==
  data: dp_aa_t input; dp_ff_t input; dp_phi_t input; dp_1 output; t input
function dp_1 = fcn(dp_aa_t, dp_ff_t, dp_phi_t, t)
%%%% 平移动力学方程中的扰动项设置
epsil_t = zeros(3, 1);

for kk = 1:5
    epsil_t = epsil_t + dp_aa_t(:, kk) .* sin( 2 * pi * dp_ff_t(:, kk) * t + dp_phi_t(:, kk) );
end

dp_1 = [ epsil_t(1) + 1.6 * sin( 0.4 * t ) + 2.0 * cos( 0.5 * t ) + 1.4 * sin( 0.7 * t ) ...
                + 4 * exp( -0.1 * t ) * sin( 0.8 * t ) + 3 / ( 1 + exp( -0.2 * ( t - 15 ) ) ); ...
                epsil_t(2) + 1.2 * sin( 0.2 * t ) + 3 * cos( 0.4 * t ) + 0.8 * sin( 0.6 * t ) ...
                + 2 * exp( -0.15 * t ) * cos( 1.2 * t ) + 3 / ( 1 + exp( -0.3 * ( t - 25 ) ) ); ...
                epsil_t(3) + 1.8 * sin( 0.2 * t ) + 1.6 * sin( 0.3 * t ) + 1.6 * cos( 0.4 * t ) ...
                + 4 * exp( -0.05 * t ) * sin( 0.5 * t + pi / 4 ) + 3 / ( 1 + exp( -0.5 * ( t - 20 ) ) ) ];

== matlab function sim_tvt_2025_pos_ctrl/cal err_pos_i agent 1 ==
  data: delta_ksi_vec input; ksi_i_vec input; ksi_ld_hat_vec input; err_pos_1 output
function err_pos_1 = fcn(delta_ksi_vec, ksi_i_vec, ksi_ld_hat_vec)
%%%% 计算基于分布式观测值的位置跟踪误差
iiuav = 1;
err_pos_1 = ksi_i_vec(:,iiuav) - ksi_ld_hat_vec(:,iiuav) - delta_ksi_vec(:,iiuav);

== matlab function sim_tvt_2025_pos_ctrl/cal err_pos_i agent 2 ==
  data: delta_ksi_vec input; ksi_i_vec input; ksi_ld_hat_vec input; err_pos_2 output
function err_pos_2 = fcn(delta_ksi_vec, ksi_i_vec, ksi_ld_hat_vec)
%%%% 计算基于分布式观测值的位置跟踪误差
iiuav = 2;
err_pos_2 = ksi_i_vec(:,iiuav) - ksi_ld_hat_vec(:,iiuav) - delta_ksi_vec(:,iiuav);

== matlab function sim_tvt_2025_pos_ctrl/cal err_pos_i agent 3 ==
  data: delta_ksi_vec input; ksi_i_vec input; ksi_ld_hat_vec input; err_pos_3 output
function err_pos_3 = fcn(delta_ksi_vec, ksi_i_vec, ksi_ld_hat_vec)
%%%% 计算基于分布式观测值的位置跟踪误差
iiuav = 3;
err_pos_3 = ksi_i_vec(:,iiuav) - ksi_ld_hat_vec(:,iiuav) - delta_ksi_vec(:,iiuav);

== matlab function sim_tvt_2025_pos_ctrl/cal err_pos_i agent 4 ==
  data: delta_ksi_vec input; ksi_i_vec input; ksi_ld_hat_vec input; err_pos_4 output
function err_pos_4 = fcn(delta_ksi_vec, ksi_i_vec, ksi_ld_hat_vec)
%%%% 计算基于分布式观测值的位置跟踪误差
iiuav = 4;
err_pos_4 = ksi_i_vec(:,iiuav) - ksi_ld_hat_vec(:,iiuav) - delta_ksi_vec(:,iiuav);

== matlab function sim_tvt_2025_pos_ctrl/cal err_pos_i agent 5 ==
  data: delta_ksi_vec input; ksi_i_vec input; ksi_ld_hat_vec input; err_pos_5 output
function err_pos_5 = fcn(delta_ksi_vec, ksi_i_vec, ksi_ld_hat_vec)
%%%% 计算基于分布式观测值的位置跟踪误差
iiuav = 5;
err_pos_5 = ksi_i_vec(:,iiuav) - ksi_ld_hat_vec(:,iiuav) - delta_ksi_vec(:,iiuav);

== matlab function sim_tvt_2025_pos_ctrl/combine err_pos_i ==
  data: err_pos_1 input; err_pos_vec output; err_pos_2 input; err_pos_3 input; err_pos_4 input; err_pos_5 input
function err_pos_vec  = fcn(err_pos_1, err_pos_2, err_pos_3, err_pos_4, err_pos_5)
%%%% 合并基于分布式观测值的位置跟踪误差
err_pos_vec = zeros(3,5);
err_pos_vec(:,1) = err_pos_1(:);
err_pos_vec(:,2) = err_pos_2(:);
err_pos_vec(:,3) = err_pos_3(:);
err_pos_vec(:,4) = err_pos_4(:);
err_pos_vec(:,5) = err_pos_5(:);

== matlab function sim_tvt_2025_pos_ctrl/cal err_vel_i agent 1 ==
  data: delta_eta_vec input; eta_i_vec input; eta_ld_hat_vec input; err_vel_1 output
function err_vel_1 = fcn(delta_eta_vec, eta_i_vec, eta_ld_hat_vec)
%%%% 计算基于分布式观测值的速度跟踪误差
iiuav = 1;
err_vel_1 = eta_i_vec(:,iiuav) - eta_ld_hat_vec(:,iiuav) - delta_eta_vec(:,iiuav);

== matlab function sim_tvt_2025_pos_ctrl/cal err_vel_i agent 2 ==
  data: delta_eta_vec input; eta_i_vec input; eta_ld_hat_vec input; err_vel_2 output
function err_vel_2 = fcn(delta_eta_vec, eta_i_vec, eta_ld_hat_vec)
%%%% 计算基于分布式观测值的速度跟踪误差
iiuav = 2;
err_vel_2 = eta_i_vec(:,iiuav) - eta_ld_hat_vec(:,iiuav) - delta_eta_vec(:,iiuav);

== matlab function sim_tvt_2025_pos_ctrl/cal err_vel_i agent 3 ==
  data: delta_eta_vec input; eta_i_vec input; eta_ld_hat_vec input; err_vel_3 output
function err_vel_3 = fcn(delta_eta_vec, eta_i_vec, eta_ld_hat_vec)
%%%% 计算基于分布式观测值的速度跟踪误差
iiuav = 3;
err_vel_3 = eta_i_vec(:,iiuav) - eta_ld_hat_vec(:,iiuav) - delta_eta_vec(:,iiuav);

== matlab function sim_tvt_2025_pos_ctrl/cal err_vel_i agent 4 ==
  data: delta_eta_vec input; eta_i_vec input; eta_ld_hat_vec input; err_vel_4 output
function err_vel_4 = fcn(delta_eta_vec, eta_i_vec, eta_ld_hat_vec)
%%%% 计算基于分布式观测值的速度跟踪误差
iiuav = 4;
err_vel_4 = eta_i_vec(:,iiuav) - eta_ld_hat_vec(:,iiuav) - delta_eta_vec(:,iiuav);

== matlab function sim_tvt_2025_pos_ctrl/cal err_vel_i agent 5 ==
  data: delta_eta_vec input; eta_i_vec input; eta_ld_hat_vec input; err_vel_5 output
function err_vel_5 = fcn(delta_eta_vec, eta_i_vec, eta_ld_hat_vec)
%%%% 计算基于分布式观测值的速度跟踪误差
iiuav = 5;
err_vel_5 = eta_i_vec(:,iiuav) - eta_ld_hat_vec(:,iiuav) - delta_eta_vec(:,iiuav);

== matlab function sim_tvt_2025_pos_ctrl/generate translational disturbance agent 2 ==
  data: dp_aa_t input; dp_ff_t input; dp_phi_t input; dp_2 output; t input
function dp_2 = fcn(dp_aa_t, dp_ff_t, dp_phi_t, t)
%%%% 平移动力学方程中的扰动项设置
epsil_t = zeros(3, 1);

for kk = 1:5
    epsil_t = epsil_t + dp_aa_t(:, kk) .* sin( 2 * pi * dp_ff_t(:, kk) * t + dp_phi_t(:, kk) );
end

dp_2 = [ epsil_t(1) + 1.6 * sin( 0.2 * t ) + 2.0 * cos( 0.3 * t ) + 1.4 * sin( 0.5 * t ) ...
                + 4 * exp( -0.1 * t ) * sin( 0.5 * t ) + 3 / ( 1 + exp( -0.2 * ( t - 15 ) ) ); ...
                epsil_t(2) + 1.2 * sin( 0.1 * t ) + 3 * cos( 0.2 * t ) + 0.8 * sin( 0.4 * t ) ...
                + 2 * exp( -0.15 * t ) * cos( 0.6 * t ) + 3 / ( 1 + exp( -0.3 * ( t - 25 ) ) ); ...
                epsil_t(3) + 1.8 * sin( 0.1 * t ) + 1.6 * sin( 0.2 * t ) + 1.6 * cos( 0.3 * t ) ...
                + 4 * exp( -0.05 * t ) * sin( 0.4 * t + pi / 4 ) + 3 / ( 1 + exp( -0.5 * ( t - 20 ) ) ) ];

== matlab function sim_tvt_2025_pos_ctrl/combine err_vel_i ==
  data: err_vel_1 input; err_vel_vec output; err_vel_2 input; err_vel_3 input; err_vel_4 input; err_vel_5 input
function err_vel_vec  = fcn(err_vel_1, err_vel_2, err_vel_3, err_vel_4, err_vel_5)
%%%% 合并基于分布式观测值的速度跟踪误差
err_vel_vec = zeros(3,5);
err_vel_vec(:,1) = err_vel_1(:);
err_vel_vec(:,2) = err_vel_2(:);
err_vel_vec(:,3) = err_vel_3(:);
err_vel_vec(:,4) = err_vel_4(:);
err_vel_vec(:,5) = err_vel_5(:);

== matlab function sim_tvt_2025_pos_ctrl/cal err_pos_bar_i agent 1 ==
  data: err_pos_vec input; phi_vec input; err_pos_bar_1 output
function err_pos_bar_1 = fcn(err_pos_vec, phi_vec)
%%%% 计算虚拟位置跟踪误差
iiuav = 1;
err_pos_bar_1 = err_pos_vec(:,iiuav) - phi_vec(:,iiuav);

== matlab function sim_tvt_2025_pos_ctrl/choose eta_est_err_tilt 12 ==
  data: x input; y output
function y = fcn(x)
iiuav = 5;
y = x(:,iiuav);

== matlab function sim_tvt_2025_pos_ctrl/choose eta_est_err_tilt 13 ==
  data: x input; y output
function y = fcn(x)
iiuav = 1;
y = x(:,iiuav);

== matlab function sim_tvt_2025_pos_ctrl/choose eta_est_err_tilt 14 ==
  data: x input; y output
function y = fcn(x)
iiuav = 2;
y = x(:,iiuav);

== matlab function sim_tvt_2025_pos_ctrl/choose eta_est_err_tilt 15 ==
  data: x input; y output
function y = fcn(x)
iiuav = 2;
y = x(:,iiuav);

== matlab function sim_tvt_2025_pos_ctrl/choose eta_est_err_tilt 16 ==
  data: x input; y output
function y = fcn(x)
iiuav = 3;
y = x(:,iiuav);

== matlab function sim_tvt_2025_pos_ctrl/choose eta_est_err_tilt 17 ==
  data: x input; y output
function y = fcn(x)
iiuav = 3;
y = x(:,iiuav);

== matlab function sim_tvt_2025_pos_ctrl/combine leader position estimaters ==
  data: ksi_d_est_1 input; ksi_d_est_vec output; ksi_d_est_2 input; ksi_d_est_3 input; ksi_d_est_4 input; ksi_d_est_5 input
function ksi_d_est_vec  = fcn(ksi_d_est_1, ksi_d_est_2, ksi_d_est_3, ksi_d_est_4, ksi_d_est_5)
%%%% 合并领导者位置观测器输出结果
ksi_d_est_vec = [ksi_d_est_1(:), ksi_d_est_2(:), ksi_d_est_3(:), ksi_d_est_4(:), ksi_d_est_5(:)];

== matlab function sim_tvt_2025_pos_ctrl/cal leader velocity observation ==
  data: eta_d_est_vec input; eta_ld_hat_vec output; delta_eta_vec input
function eta_ld_hat_vec  = fcn(eta_d_est_vec, delta_eta_vec)
%%%% 计算领导者期望速度观测值
eta_ld_hat_vec = zeros(3,5);
for iiuav = 1:5
    eta_ld_hat_vec(:,iiuav) = eta_d_est_vec(:,iiuav) - delta_eta_vec(:,iiuav);
end

== matlab function sim_tvt_2025_pos_ctrl/cal leader position observation ==
  data: ksi_d_est_vec input; ksi_ld_hat_vec output; delta_ksi_vec input
function ksi_ld_hat_vec  = fcn(ksi_d_est_vec, delta_ksi_vec)
%%%% 计算领导者期望速度观测值
ksi_ld_hat_vec = zeros(3,5);
for iiuav = 1:5
    ksi_ld_hat_vec(:,iiuav) = ksi_d_est_vec(:,iiuav) - delta_ksi_vec(:,iiuav);
end

== matlab function sim_tvt_2025_pos_ctrl/cal err_pos_bar_i agent 2 ==
  data: err_pos_vec input; phi_vec input; err_pos_bar_2 output
function err_pos_bar_2 = fcn(err_pos_vec, phi_vec)
%%%% 计算虚拟位置跟踪误差
iiuav = 2;
err_pos_bar_2 = err_pos_vec(:,iiuav) - phi_vec(:,iiuav);

== matlab function sim_tvt_2025_pos_ctrl/generate translational disturbance agent 3 ==
  data: dp_aa_t input; dp_ff_t input; dp_phi_t input; dp_3 output; t input
function dp_3 = fcn(dp_aa_t, dp_ff_t, dp_phi_t, t)
%%%% 平移动力学方程中的扰动项设置
epsil_t = zeros(3, 1);

for kk = 1:5
    epsil_t = epsil_t + dp_aa_t(:, kk) .* sin( 2 * pi * dp_ff_t(:, kk) * t + dp_phi_t(:, kk) );
end

dp_3 = [ epsil_t(1) + 1.6 * sin( 0.2 * t ) + 2.0 * cos( 0.3 * t ) + 1.4 * sin( 0.5 * t ) ...
                + 4 * exp( -0.1 * t ) * sin( 0.5 * t ) + 3 / ( 1 + exp( -0.2 * ( t - 15 ) ) ); ...
                epsil_t(2) + 1.2 * sin( 0.1 * t ) + 3 * cos( 0.2 * t ) + 0.8 * sin( 0.4 * t ) ...
                + 2 * exp( -0.15 * t ) * cos( 0.6 * t ) + 3 / ( 1 + exp( -0.3 * ( t - 25 ) ) ); ...
                epsil_t(3) + 1.8 * sin( 0.1 * t ) + 1.6 * sin( 0.2 * t ) + 1.6 * cos( 0.3 * t ) ...
                + 4 * exp( -0.05 * t ) * sin( 0.4 * t + pi / 4 ) + 3 / ( 1 + exp( -0.5 * ( t - 20 ) ) ) ];

== matlab function sim_tvt_2025_pos_ctrl/cal err_pos_bar_i agent 3 ==
  data: err_pos_vec input; phi_vec input; err_pos_bar_3 output
function err_pos_bar_3 = fcn(err_pos_vec, phi_vec)
%%%% 计算虚拟位置跟踪误差
iiuav = 3;
err_pos_bar_3 = err_pos_vec(:,iiuav) - phi_vec(:,iiuav);

== matlab function sim_tvt_2025_pos_ctrl/cal err_pos_bar_i agent 4 ==
  data: err_pos_vec input; phi_vec input; err_pos_bar_4 output
function err_pos_bar_4 = fcn(err_pos_vec, phi_vec)
%%%% 计算虚拟位置跟踪误差
iiuav = 4;
err_pos_bar_4 = err_pos_vec(:,iiuav) - phi_vec(:,iiuav);

== matlab function sim_tvt_2025_pos_ctrl/cal err_pos_bar_i agent 5 ==
  data: err_pos_vec input; phi_vec input; err_pos_bar_5 output
function err_pos_bar_5 = fcn(err_pos_vec, phi_vec)
%%%% 计算虚拟位置跟踪误差
iiuav = 5;
err_pos_bar_5 = err_pos_vec(:,iiuav) - phi_vec(:,iiuav);

== matlab function sim_tvt_2025_pos_ctrl/combine err_pos_bar_i ==
  data: err_pos_bar_1 input; err_pos_bar_vec output; err_pos_bar_2 input; err_pos_bar_3 input; err_pos_bar_4 input; err_pos_bar_5 input
function err_pos_bar_vec  = fcn(err_pos_bar_1, err_pos_bar_2, err_pos_bar_3, err_pos_bar_4, err_pos_bar_5)
%%%% 合并虚拟位置跟踪误差
err_pos_bar_vec = zeros(3,5);
err_pos_bar_vec(:,1) = err_pos_bar_1(:);
err_pos_bar_vec(:,2) = err_pos_bar_2(:);
err_pos_bar_vec(:,3) = err_pos_bar_3(:);
err_pos_bar_vec(:,4) = err_pos_bar_4(:);
err_pos_bar_vec(:,5) = err_pos_bar_5(:);

== matlab function sim_tvt_2025_pos_ctrl/cal err_vel_bar_i agent 1 ==
  data: err_vel_vec input; d_phi_vec input; err_vel_bar_1 output
function err_vel_bar_1 = fcn(err_vel_vec, d_phi_vec)
%%%% 计算虚拟速度跟踪误差
iiuav = 1;
err_vel_bar_1 = err_vel_vec(:,iiuav) - d_phi_vec(:,iiuav);

== matlab function sim_tvt_2025_pos_ctrl/cal err_vel_bar_i agent 2 ==
  data: err_vel_vec input; d_phi_vec input; err_vel_bar_2 output
function err_vel_bar_2 = fcn(err_vel_vec, d_phi_vec)
%%%% 计算虚拟速度跟踪误差
iiuav = 2;
err_vel_bar_2 = err_vel_vec(:,iiuav) - d_phi_vec(:,iiuav);
